simulink model "PID_controller_simulation"  (Simulink 7.3)
settings: Solver=ode45  StartTime=0.0  StopTime=300  RelTol=1e-3
libraries: powerlib_extras x1, gauges_gmslib x1
settings Model: Creator=cheidelb  LastModifiedBy=cheidelb

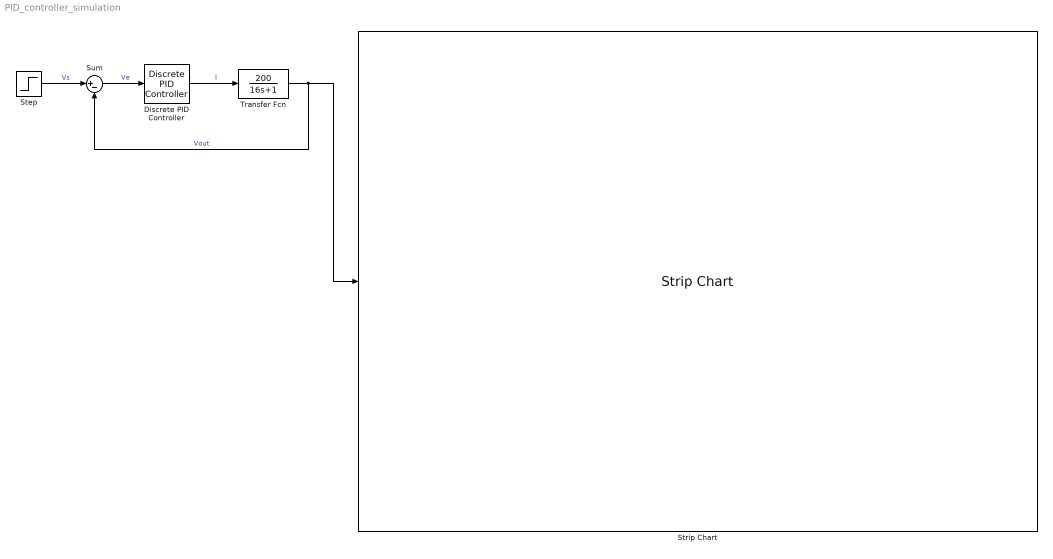
== system PID_controller_simulation ==
  Discrete PID Controller : powerlib_extras/Discrete  Control Blocks/Discrete PID Controller  DialogController=POWERSYS.PowerSysDialog  SystemSampleTime=-1  Kp=.002  Ki=.000333  Kd=.0003  TcD=1  Par_Limits=[10 0]  Init=0  Ts=.5
  Step : Step  After=400  SampleTime=0
  Strip Chart : gauges_gmslib/Strip Chart/Strip Chart  progid=mwStrip.stripctrl.1  connect=input  init="hActx.XTicMode = 1;hActx.XSpan = 10/60/60/24; hActx.TimeSecondsFormat = '%M:%S'; hActx.TimeDateFormat = ''; hActx.TimeDaysFormat = ''; hActx.TimeHoursFormat = ''; hActx.TimeMinutesFormat = ''; hActx.TimeMonthsFormat = ''; hActx.TimeYearsFormat = ''; % Set x-axis to display time; set span = 10 sec (in fixed units=days); set display format = \"min:sec\" only"  inblock=on  border=on  updateParam=0
  Sum : Sum  Inputs=|+-  OutDataType=fixdt(1, 16)  OutScaling=2^0
  Transfer Fcn : TransferFcn  Numerator=[200]  Denominator=[16 1]
  wires:
  Sum/1 -> Discrete PID Controller/1  "Ve"
  Discrete PID Controller/1 -> Transfer Fcn/1  "I"
  Transfer Fcn/1 -> Strip Chart/1, Sum/2  "Vout"
  Step/1 -> Sum/1  "Vs"
